simulink model "ControlePreditivoSala"  (R2017b)
settings: Solver=VariableStepAuto  StartTime=0.0  StopTime=10.0  RelTol=1e-3
libraries: embdlinuxlib x1
settings Model: Creator=heyderaraujo  LastModifiedBy=heyderaraujo

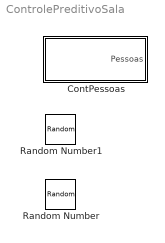
== system ControlePreditivoSala ==
  ContPessoas : Subsystem
  Random Number : RandomNumber  Variance=2.5  Seed=23  SampleTime=0.1
  Random Number1 : RandomNumber  Variance=2.5  Seed=28  SampleTime=0.1

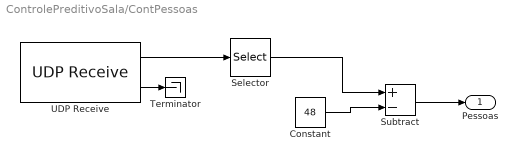
== system ControlePreditivoSala/ContPessoas ==
  Constant : Constant  Value=48
  Selector : Selector  InputPortWidth=255  IndexOptions=Starting index (dialog)  Indices=[1]  OutputSizes=1
  Subtract : Sum  Inputs=+-
  Terminator : Terminator
  UDP Receive : embdlinuxlib/UDP Receive  localURL='0.0.0.0'  localPort=625  remoteURL='0.0.0.0'  remotePort=-1  recvBufferSize=8192  signalDatatype=uint8  dims=255  isVarSize=off  showBlockingTime=off  blockingTime=0  sampletime=0.01  blockPlatform=Raspberry Pi
      settings: SourceProductName=Simulink Support Package for Raspberry Pi Hardware  SourceProductBaseCode=RASPPI
  "Pessoas " : Outport
  wires:
  Selector/1 -> Subtract/1
  UDP Receive/1 -> Selector/1
  Constant/1 -> Subtract/2
  Subtract/1 -> "Pessoas "/1
  UDP Receive/2 -> Terminator/1
